simulink model "Udan_SOC"  (R2017b)
settings: Solver=FixedStepAuto  StartTime=0.0  StopTime=1000  FixedStep=0.1  RelTol=1e-3
values from neighbouring files (symbols this model uses):
  DenominatorOfIntegratorFactor = 100.0    [SOC_Stateflow.sldd]
  SOC_CalcSohLKT = 1.0    [SOC_Stateflow.sldd]
  SOC_CalcSOHTempLimit = 70.0    [SOC_Stateflow.sldd]
  SOC_CapPerCycle = 100.0    [SOC_Stateflow.sldd]
  SOC_CapTemp_HLimit = 200.0    [SOC_Stateflow.sldd]
  SOC_CapTemp_LLimit = 0.0    [SOC_Stateflow.sldd]
  Soc_ConfigInfo = 0    [SOC_Stateflow.sldd]
  SOC_DchgEndCalib = 0.0    [SOC_Stateflow.sldd]
  SOC_DiffVoltMin = 10.0    [SOC_Stateflow.sldd]
  SOC_DSOCJumpMax = 500.0    [SOC_Stateflow.sldd]
  SOC_EfficientHighLimit = 250.0    [SOC_Stateflow.sldd]
  SOC_EfficientLowLimit = 40.0    [SOC_Stateflow.sldd]
  SOC_EmptyAus = 0.0    [SOC_Stateflow.sldd]
  SOC_EnableOcv = 1.0    [SOC_Stateflow.sldd]
  SOC_END_CALIB_STATE : value not decoded    [SOC_Stateflow.sldd]
  SOC_HighRealSoc = 95.0    [SOC_Stateflow.sldd]
  SOC_LKTSohCycles = 0.0 1.0 10.0 20.0 30.0 40.0 50.0 60.0 70.0 80.0 90.0 100.0 110.0 120.0 130.0 140.0 150.0 160.0 170.0 180.0 190.0 200.0 210.0 220.0 230.0 240.0 250.0 260.0 270.0 280.0 290.0 300.0 310.0 320.0 330.0 340.0 350.0 360.0 370.0 380.0 390.0 400.0 410.0 420.0 430.0 440.0 450.0 460.0 470.0 480.0 490.0 500.0 510.0 520.0 530.0 540.0 550.0 560.0 570.0 580.0 590.0 600.0 610.0 620.0 630.0 640.0 650.0 660.0 670.0    [SOC_Stateflow.sldd]
  SOC_LKTSohTable = 1000.0 991.0 989.0 992.0 993.0 995.0 994.0 993.0 1000.0 997.0 1002.0 1000.0 992.0 1000.0 989.0 992.0 989.0 994.0 989.0 993.0 994.0 994.0 994.0 993.0 991.0 991.0 992.0 993.0 991.0 985.0 985.0 985.0 979.0 975.0 978.0 984.0 982.0 974.0 975.0 972.0 972.0 975.0 977.0 977.0 974.0 971.0 973.0 971.0 966.0 968.0 965.0 959.0 957.0 956.0 957.0 954.0 955.0 951.0 954.0 951.0 942.0 942.0 940.0 942.0 947.0 949.0    [SOC_Stateflow.sldd]
  SOC_LowRealSoc = 5.0    [SOC_Stateflow.sldd]
  SOC_NominalCap_AmS = 576000000.0    [SOC_Stateflow.sldd]
  SOC_NominalVol = 4000.0    [SOC_Stateflow.sldd]
  SOC_OCVTemp_HLimit = 106.0    [SOC_Stateflow.sldd]
  SOC_OCVTemp_LLimit = 29.0    [SOC_Stateflow.sldd]
  SOC_ShortCalibDSoc = 1.0    [SOC_Stateflow.sldd]
  SOC_SOCResolution = 10000.0    [SOC_Stateflow.sldd]
  SOC_SohCalcCapPercent = 8.0    [SOC_Stateflow.sldd]
  SOC_SohCalcHighLimit = 60.0    [SOC_Stateflow.sldd]
  SOC_SohCalcLowLimit = 10.0    [SOC_Stateflow.sldd]
  SOC_SohCalcMidLimit = 30.0    [SOC_Stateflow.sldd]
  SOC_SOHResolution = 1000.0    [SOC_Stateflow.sldd]
  SOC_State = <binary blob, 1163 chars, not shown>    [SOC_Stateflow.sldd]
  SOC_TempCap_CapBuffer : value not decoded    [SOC_Stateflow.sldd]
  SOC_TempCap_TempBuffer : value not decoded    [SOC_Stateflow.sldd]
  SocOcvCalib_ConfigInfo = 0.0    [SOC_Stateflow.sldd]
  SocOcvCalib_SocBuffer1 : value not decoded    [SOC_Stateflow.sldd]
  SocOcvCalib_TempBuffer : value not decoded    [SOC_Stateflow.sldd]
  SocOcvCalib_VoltageBuffer1 = 3300.0 3303.0 3305.0 3307.0 3310.0 3311.0 3313.0 3314.0 3316.0 3317.0 3319.0 3320.0 3322.0 3323.0 3325.0 3322.0 3323.0 3325.0 3310.0 3313.0 3315.0 3317.0 3320.0 3321.0 3323.0 3324.0 3326.0 3327.0 3329.0 3330.0 3332.0 3333.0 3335.0 3332.0 3333.0 3335.0 3320.0 3323.0 3325.0 3327.0 3330.0 3331.0 3333.0 3334.0 3336.0 3337.0 3339.0 3340.0 3342.0 3343.0 3345.0 3342.0 3343.0 3345.0 3330.0 3333.0 3335.0 3    [SOC_Stateflow.sldd]
  SOHCalibCycle = 10.0    [SOC_Stateflow.sldd]
undefined symbols (not defined in the file or in its folder): DatetimeM_GetReturnType, ParameterM_EeepParaIndexType, Soc_CumuLativeTypeType, SOC_EgthTempChgValue, Soc_EnergyBuffer, SOC_FithTempChgValue, SOC_FstSlowTempChgValue, SOC_FstTempChgValue, SOC_FthTempChgValue, SOC_MaxCap_AmS, SOC_SethTempChgValue, SOC_SixTempChgValue, SOC_SndSlowTempChgValue, SOC_SndTempChgValue, SOC_TrdSlowTempChgValue, SOC_TrdTempChgValue, SocDiagCalib_NoCalibReasonType
libraries: simulink x138, hdlsllib x24, dspindex x4
(part 7 of 10)

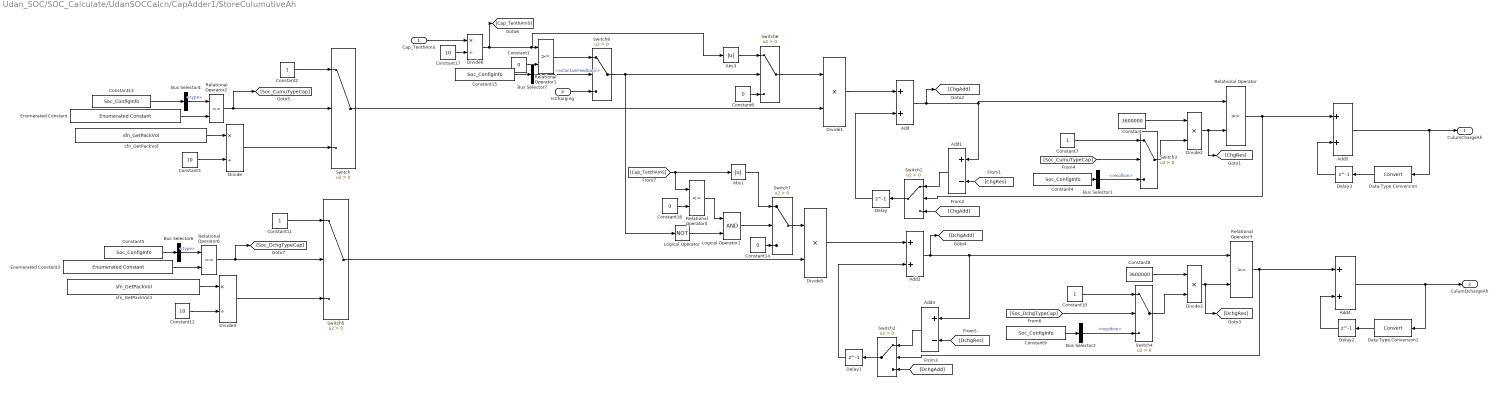
== system Udan_SOC/SOC_Calculate/UdanSOCCalcn/CapAdder1/StoreCulumutiveAh ==
  Cap_TenthAmS : Inport
  IsCharging : Inport  Port=2
  Abs1 : Abs
  Abs3 : Abs
  Add : Sum  OutDataTypeStr=uint32
  Add1 : Sum  Inputs=+-  OutDataTypeStr=int32
  Add2 : Sum  OutDataTypeStr=uint32
  Add3 : Sum  Inputs=+-  OutDataTypeStr=int32
  Add4 : Sum
  Add5 : Sum
  Bus Selector1 : BusSelector  OutputSignals=ChgCumuInfo.resoltion
  Bus Selector2 : BusSelector  OutputSignals=DchgCumuInfo.resoltion
  Bus Selector4 : BusSelector  OutputSignals=ChgCumuInfo.type
  Bus Selector6 : BusSelector  OutputSignals=DchgCumuInfo.type
  Bus Selector7 : BusSelector  OutputSignals=ChgCumuInfo.isContainFeedback
  Constant : Constant  Value=3600000  OutDataTypeStr=uint32
  Constant{1,6,14,16} (4 alike) : Constant  Value=0  OutDataTypeStr=uint8
  Constant{2,7,10..11} (4 alike) : Constant  OutDataTypeStr=uint16
  Constant12 : Constant  Value=10  OutDataTypeStr=uint8
  Constant{4..5,9,13,15} (5 alike) : Constant  Value=Soc_ConfigInfo  OutDataTypeStr=Bus: Soc_ConfigInfoType
  Constant17 : Constant  Value=10  OutDataTypeStr=uint8
  Constant3 : Constant  Value=10  OutDataTypeStr=uint8
  Constant8 : Constant  Value=3600000  OutDataTypeStr=uint32
  Data Type Conversion : DataTypeConversion
  Data Type Conversion1 : DataTypeConversion
  Delay{,1..3} (4 alike) : Delay  DelayLength=1  InitialCondition=0
  Divide : Product  Inputs=*/  OutDataTypeStr=uint16
  Divide{1..3,5} (4 alike) : Product  Inputs=**  OutDataTypeStr=uint32
  Divide4 : Product  Inputs=*/  OutDataTypeStr=uint16
  Divide6 : Product  Inputs=*/  OutDataTypeStr=int32
  Enumerated Constant : simulink/Sources/Enumerated Constant  OutDataTypeStr=Enum: Soc_CumuLativeTypeType  Value=Soc_CumuLativeTypeType.Soc_CumuTypeCap  SampleTime=inf
      settings: SourceProductName=Simulink
  Enumerated Constant3 : simulink/Sources/Enumerated Constant  OutDataTypeStr=Enum: Soc_CumuLativeTypeType  Value=Soc_CumuLativeTypeType.Soc_CumuTypeCap  SampleTime=inf
      settings: SourceProductName=Simulink
  Logical Operator : Logic  Operator=NOT  AllPortsSameDT=off  OutDataTypeStr=boolean
  Logical Operator1 : Logic  AllPortsSameDT=off  OutDataTypeStr=boolean
  Relational Operator : RelationalOperator  OutDataTypeStr=boolean  RndMeth=Simplest
  Relational Operator1 : RelationalOperator  OutDataTypeStr=boolean  RndMeth=Simplest
  Relational Operator2 : RelationalOperator  Operator===  OutDataTypeStr=boolean  RndMeth=Simplest
  Relational Operator3 : RelationalOperator  OutDataTypeStr=boolean  RndMeth=Simplest
  Relational Operator4 : RelationalOperator  Operator=<=  OutDataTypeStr=boolean  RndMeth=Simplest
  Relational Operator6 : RelationalOperator  Operator===  OutDataTypeStr=boolean  RndMeth=Simplest
  Switch{,1..2,5,8} (5 alike) : Switch  Criteria=u2 > Threshold
  Switch3 : Switch  Criteria=u2 > Threshold  OutDataTypeStr=uint16
  Switch4 : Switch  Criteria=u2 > Threshold  OutDataTypeStr=uint16
  Switch6 : Switch  Criteria=u2 > Threshold  OutDataTypeStr=uint32
  Switch7 : Switch  Criteria=u2 > Threshold  OutDataTypeStr=int32
  sfn_GetPackVol : S-Function  FunctionName=sfn_GetPackVol  SFunctionDeploymentMode=off  EnableBusSupport=off  mask(Legacy Function){SFunctionSpec=uint16 y1=Statistic_GetBcu100mvTotalVoltage(void), ShowSpec=on}
      mask prompts: ShowSpec "Display function specification"
      mask help:
      | This block allows you to call the legacy functions specified by the following Legacy Code Tool definition:
      | def.SFunctionName = 'sfn_GetPackVol';
      | def.OutputFcnSpec = 'uint16 y1=Statistic_GetBcu100mvTotalVoltage(void)';
      | def.HeaderFiles = {'Statistic.h'};
      mask Help: <p>This block was generated automatically by the Legacy Code Tool. For detailed help on this tool, call<a href="matlab:legacy_code('help')"> legacy_code('help')</a>.</p>
      mask Callback ShowSpec:
      | if strcmp(get_param(gcbh, 'ShowSpec'), 'on')
      |   set_param(gcbh, 'MaskDisplay', sprintf('fprintf(''%s'');', get_param(gcbh, 'SFunctionSpec')));
      | else
      |   set_param(gcbh, 'MaskDisplay', sprintf('fprintf(''%s'');', get_param(gcbh, 'FunctionName')));
      | end
      mask Display: fprintf('uint16 y1=Statistic_GetBcu100mvTotalVoltage(void)');
  sfn_GetPackVol1 : S-Function  FunctionName=sfn_GetPackVol  SFunctionDeploymentMode=off  EnableBusSupport=off  mask(Legacy Function){SFunctionSpec=uint16 y1=Statistic_GetBcu100mvTotalVoltage(void), ShowSpec=on}
      mask prompts: ShowSpec "Display function specification"
      mask help:
      | This block allows you to call the legacy functions specified by the following Legacy Code Tool definition:
      | def.SFunctionName = 'sfn_GetPackVol';
      | def.OutputFcnSpec = 'uint16 y1=Statistic_GetBcu100mvTotalVoltage(void)';
      | def.HeaderFiles = {'Statistic.h'};
      mask Help: <p>This block was generated automatically by the Legacy Code Tool. For detailed help on this tool, call<a href="matlab:legacy_code('help')"> legacy_code('help')</a>.</p>
      mask Callback ShowSpec:
      | if strcmp(get_param(gcbh, 'ShowSpec'), 'on')
      |   set_param(gcbh, 'MaskDisplay', sprintf('fprintf(''%s'');', get_param(gcbh, 'SFunctionSpec')));
      | else
      |   set_param(gcbh, 'MaskDisplay', sprintf('fprintf(''%s'');', get_param(gcbh, 'FunctionName')));
      | end
      mask Display: fprintf('uint16 y1=Statistic_GetBcu100mvTotalVoltage(void)');
  CulumChargeAh : Outport
  CulumDchargeAh : Outport  Port=2
  wires:
  Data Type Conversion1/1 -> Delay2/1
  Data Type Conversion/1 -> Delay3/1
  Divide1/1 -> Add/1
  Add2/1 -> [DchgAdd], Add3/1, Relational Operator3/1
  Delay1/1 -> Add2/2
  [DchgRes] -> Add3/2
  Switch2/1 -> Delay1/1
  [DchgAdd] -> Switch2/3
  Add3/1 -> Switch2/1
  Delay/1 -> Add/2
  [ChgAdd] -> Switch1/3
  Add1/1 -> Switch1/1
  [ChgRes] -> Add1/2
  Divide3/1 -> Relational Operator3/2, [DchgRes]
  Divide2/1 -> [ChgRes], Relational Operator/2
  Constant4/1 -> Bus Selector1/1
  Bus Selector1/1 -> Switch3/3  "<resoltion>"
  Switch/1 -> Divide1/2
  Divide6/1 -> Relational Operator1/1, Abs3/1, [Cap_TenthAmS]
  Divide/1 -> Switch/3
  Constant3/1 -> Divide/2
  sfn_GetPackVol/1 -> Divide/1
  Constant2/1 -> Switch/1
  Relational Operator2/1 -> Switch/2, [Soc_CumuTypeCap]
  Enumerated Constant/1 -> Relational Operator2/2
  Constant13/1 -> Bus Selector4/1
  Bus Selector4/1 -> Relational Operator2/1  "<type>"
  Constant/1 -> Divide2/1
  Add/1 -> Add1/1, Relational Operator/1, [ChgAdd]
  Switch1/1 -> Delay/1
  [Soc_CumuTypeCap] -> Switch3/2
  Constant7/1 -> Switch3/1
  Switch3/1 -> Divide2/2
  Switch4/1 -> Divide3/2
  Bus Selector2/1 -> Switch4/3  "<resoltion>"
  Constant9/1 -> Bus Selector2/1
  Constant8/1 -> Divide3/1
  [Soc_DchgTypeCap] -> Switch4/2
  Constant10/1 -> Switch4/1
  Constant11/1 -> Switch5/1
  Relational Operator6/1 -> [Soc_DchgTypeCap], Switch5/2
  Constant5/1 -> Bus Selector6/1
  Enumerated Constant3/1 -> Relational Operator6/2
  Bus Selector6/1 -> Relational Operator6/1  "<type>"
  Constant12/1 -> Divide4/2
  Divide4/1 -> Switch5/3
  sfn_GetPackVol1/1 -> Divide4/1
  [Cap_TenthAmS] -> Relational Operator4/1, Abs1/1
  Switch5/1 -> Divide5/2
  Divide5/1 -> Add2/1
  Abs1/1 -> Switch7/1
  Relational Operator3/1 -> Add4/1, Switch2/2
  IsCharging/1 -> Switch8/3
  Constant1/1 -> Relational Operator1/2
  Switch8/1 -> Switch6/2, Logical Operator/1
  Switch6/1 -> Divide1/1
  Constant6/1 -> Switch6/3
  Switch7/1 -> Divide5/1
  Logical Operator/1 -> Logical Operator1/2
  Constant14/1 -> Switch7/3
  Abs3/1 -> Switch6/1
  Add4/1 -> CulumDchargeAh/1, Data Type Conversion1/1
  Delay2/1 -> Add4/2
  Relational Operator/1 -> Add5/1, Switch1/2
  Add5/1 -> CulumChargeAh/1, Data Type Conversion/1
  Delay3/1 -> Add5/2
  Constant17/1 -> Divide6/2
  Cap_TenthAmS/1 -> Divide6/1
  Bus Selector7/1 -> Switch8/2  "<isContainFeedback>"
  Constant15/1 -> Bus Selector7/1
  Relational Operator1/1 -> Switch8/1
  Constant16/1 -> Relational Operator4/2
  Logical Operator1/1 -> Switch7/2
  Relational Operator4/1 -> Logical Operator1/1

== system Udan_SOC/SOC_Calculate/UdanSOCCalcn/CapAdder2/Function-Call Subsystem ==
  DLeftCapIn : Inport
  function : TriggerPort  VariantControl=Variant
  DLeftCapOut : Outport
  wires:
  DLeftCapIn/1 -> DLeftCapOut/1

== system Udan_SOC/SOC_Calculate/UdanSOCCalcn/ClearLeftCapWOCalib/Subsystem ==
  data : Inport
  HighIndex : Inport  Port=2
  LowIndex : Inport  Port=3
  Bit Rotate : hdlsllib/Logic and Bit Operations/Bit Rotate  mode=Rotate Right  N=16
      settings: SourceProductName=HDL Coder  SourceProductBaseCode=HD
  Data Type Conversion : DataTypeConversion  OutDataTypeStr=uint16
  Data Type Conversion1 : DataTypeConversion  OutDataTypeStr=uint16
  S-Function : S-Function  FunctionName=sfn_NVMWrite  SFunctionDeploymentMode=off  EnableBusSupport=off
  S-Function1 : S-Function  FunctionName=sfn_NVMWrite  SFunctionDeploymentMode=off  EnableBusSupport=off
  Terminator : Terminator
  Terminator1 : Terminator
  wires:
  data/1 -> Data Type Conversion1/1, Bit Rotate/1
  Data Type Conversion/1 -> S-Function/2
  S-Function1/1 -> Terminator1/1
  Bit Rotate/1 -> Data Type Conversion/1
  Data Type Conversion1/1 -> S-Function1/2
  S-Function/1 -> Terminator/1
  HighIndex/1 -> S-Function/1
  LowIndex/1 -> S-Function1/1

== system Udan_SOC/SOC_Calculate/UdanSOCCalcn/ClearLeftCapWOCalib2/Subsystem ==
  data : Inport
  HighIndex : Inport  Port=2
  LowIndex : Inport  Port=3
  Bit Rotate : hdlsllib/Logic and Bit Operations/Bit Rotate  mode=Rotate Right  N=16
      settings: SourceProductName=HDL Coder  SourceProductBaseCode=HD
  Data Type Conversion : DataTypeConversion  OutDataTypeStr=uint16
  Data Type Conversion1 : DataTypeConversion  OutDataTypeStr=uint16
  S-Function : S-Function  FunctionName=sfn_NVMWrite  SFunctionDeploymentMode=off  EnableBusSupport=off
  S-Function1 : S-Function  FunctionName=sfn_NVMWrite  SFunctionDeploymentMode=off  EnableBusSupport=off
  Terminator : Terminator
  Terminator1 : Terminator
  wires:
  data/1 -> Data Type Conversion1/1, Bit Rotate/1
  Data Type Conversion/1 -> S-Function/2
  S-Function1/1 -> Terminator1/1
  Bit Rotate/1 -> Data Type Conversion/1
  Data Type Conversion1/1 -> S-Function1/2
  S-Function/1 -> Terminator/1
  HighIndex/1 -> S-Function/1
  LowIndex/1 -> S-Function1/1

== system Udan_SOC/SOC_Calculate/UdanSOCCalcn/Function-Call Subsystem/Subsystem ==
  data : Inport
  HighIndex : Inport  Port=2
  LowIndex : Inport  Port=3
  Bit Rotate : hdlsllib/Logic and Bit Operations/Bit Rotate  mode=Rotate Right  N=16
      settings: SourceProductName=HDL Coder  SourceProductBaseCode=HD
  Data Type Conversion : DataTypeConversion  OutDataTypeStr=uint16
  Data Type Conversion1 : DataTypeConversion  OutDataTypeStr=uint16
  S-Function : S-Function  FunctionName=sfn_NVMWrite  SFunctionDeploymentMode=off  EnableBusSupport=off
  S-Function1 : S-Function  FunctionName=sfn_NVMWrite  SFunctionDeploymentMode=off  EnableBusSupport=off
  Terminator : Terminator
  Terminator1 : Terminator
  wires:
  data/1 -> Data Type Conversion1/1, Bit Rotate/1
  Data Type Conversion/1 -> S-Function/2
  S-Function1/1 -> Terminator1/1
  Bit Rotate/1 -> Data Type Conversion/1
  Data Type Conversion1/1 -> S-Function1/2
  S-Function/1 -> Terminator/1
  HighIndex/1 -> S-Function/1
  LowIndex/1 -> S-Function1/1

== system Udan_SOC/SOC_Calculate/UdanSOCCalcn/Function-Call Subsystem4/Enabled Subsystem ==
  Index : Inport
  RealSoc : Inport  Port=2
  Enable : EnablePort
  S-Function1 : S-Function  FunctionName=sfn_NVMRead  SFunctionDeploymentMode=off  EnableBusSupport=off
  Switch : Switch  Criteria=u2 > Threshold
  ReadDsocAgain : Outport
  wires:
  Index/1 -> S-Function1/1
  S-Function1/1 -> Switch/2
  RealSoc/1 -> Switch/1
  S-Function1/2 -> Switch/3
  Switch/1 -> ReadDsocAgain/1

== system Udan_SOC/SOC_Calculate/UdanSOCCalcn/Function-Call Subsystem4/Enabled Subsystem1 ==
  Enable : EnablePort
  Constant2 : Constant  Value=0  OutDataTypeStr=uint8
  Constant4 : Constant  Value=SOC_SOHResolution  OutDataTypeStr=uint16
  Enumerated Constant2 : simulink/Sources/Enumerated Constant  OutDataTypeStr=Enum: ParameterM_EeepParaIndexType  Value=ParameterM_EeepParaIndexType.PARAMETERM_EEEP_SOH_INDEX  SampleTime=inf
      settings: SourceProductName=Simulink
  Relational Operator1 : RelationalOperator  Operator=~=  OutDataTypeStr=boolean  RndMeth=Simplest
  S-Function : S-Function  FunctionName=sfn_NVMRead  SFunctionDeploymentMode=off  EnableBusSupport=off
  Switch : Switch  Criteria=u2 > Threshold
  ReadAgain : Outport
  wires:
  Enumerated Constant2/1 -> S-Function/1
  Constant2/1 -> Relational Operator1/2
  S-Function/1 -> Relational Operator1/1
  Relational Operator1/1 -> Switch/2
  S-Function/2 -> Switch/3
  Switch/1 -> ReadAgain/1
  Constant4/1 -> Switch/1

== system Udan_SOC/SOC_Calculate/UdanSOCCalcn/Function-Call Subsystem4/Subsystem1 ==
  HighIndex : Inport
  LowIndex : Inport  Port=2
  DefaultValue : Inport  Port=3
  Constant1 : Constant  Value=0  OutDataTypeStr=uint8
  Constant2 : Constant  Value=0  OutDataTypeStr=uint8
  Logical Operator : Logic  AllPortsSameDT=off  OutDataTypeStr=boolean
  Logical Operator1 : Logic  Operator=NOT  AllPortsSameDT=off  OutDataTypeStr=boolean
  Relational Operator : RelationalOperator  Operator===  OutDataTypeStr=boolean  RndMeth=Simplest
  Relational Operator1 : RelationalOperator  Operator===  OutDataTypeStr=boolean  RndMeth=Simplest
  S-Function : S-Function  FunctionName=sfn_NVMRead  SFunctionDeploymentMode=off  EnableBusSupport=off
  S-Function1 : S-Function  FunctionName=sfn_NVMRead  SFunctionDeploymentMode=off  EnableBusSupport=off
  Subsystem : Subsystem
  Subsystem1 : Subsystem  mask(ReadEeep_uint32){}
  Switch : Switch  Criteria=u2 > Threshold
  EeepRead32 : Outport
  wires:
  DefaultValue/1 -> Subsystem1/3(DefaultValue)
  [ReadLowOk] -> Logical Operator/1
  S-Function/2 -> Subsystem/1(HighIndex)
  S-Function/1 -> Relational Operator/1
  S-Function1/2 -> Subsystem/2(LowIndex)
  HighIndex/1 -> [HighIndex], S-Function/1
  Constant1/1 -> Relational Operator/2
  Constant2/1 -> Relational Operator1/2
  LowIndex/1 -> [LowIndex], S-Function1/1
  Relational Operator/1 -> Logical Operator/2
  Logical Operator/1 -> Subsystem/Enable, Logical Operator1/1
  Relational Operator1/1 -> [ReadLowOk]
  S-Function1/1 -> Relational Operator1/1
  Subsystem/1(soc) -> Switch/3
  Switch/1 -> EeepRead32/1
  [HighIndex] -> Subsystem1/1(HighIndex)
  [LowIndex] -> Subsystem1/2(LowIndex)
  Logical Operator1/1 -> [Enable], Subsystem1/Enable
  Subsystem1/1(EeepRead32) -> Switch/1
  [Enable] -> Switch/2

== system Udan_SOC/SOC_Calculate/UdanSOCCalcn/Function-Call Subsystem4/Subsystem2 ==
  SOH : Inport
  Enable : EnablePort
  Bus Selector2 : BusSelector  OutputSignals=DchgCumuInfo.resoltion
  Bus Selector4 : BusSelector  OutputSignals=DchgCumuInfo.type
  Constant : Constant  Value=SOC_LKTSohTable  VectorParams1D=off
  Constant1 : Constant  Value=SOC_LKTSohCycles  VectorParams1D=off
  Constant16 : Constant  Value=SOC_NominalCap_AmS
  Constant17 : Constant  Value=3600000  OutDataTypeStr=uint32
  Constant25 : Constant  Value=Soc_ConfigInfo  OutDataTypeStr=Bus: Soc_ConfigInfoType
  Constant26 : Constant  Value=10  OutDataTypeStr=uint8
  Constant27 : Constant  Value=Soc_ConfigInfo  OutDataTypeStr=Bus: Soc_ConfigInfoType
  Constant28 : Constant  Value=SOC_NominalVol
  Constant29 : Constant  Value=SOC_NominalCap_AmS
  Constant30 : Constant  Value=3600000  OutDataTypeStr=uint32
  Constant31 : Constant  Value=SOC_CapPerCycle  OutDataTypeStr=uint8
  Constant32 : Constant  Value=100  OutDataTypeStr=uint8
  Constant4 : Constant  Value=SOC_CapPerCycle  OutDataTypeStr=uint8
  Constant5 : Constant  Value=100  OutDataTypeStr=uint8
  DchgPower1 : simulink/Sources/Enumerated Constant  OutDataTypeStr=Enum: ParameterM_EeepParaIndexType  Value=ParameterM_EeepParaIndexType.PARAMETERM_EEEP_CUMULATIVE_DCHG_CAP_L_INDEX  SampleTime=inf
      settings: SourceProductName=Simulink
  DchgPower2 : simulink/Sources/Enumerated Constant  OutDataTypeStr=Enum: ParameterM_EeepParaIndexType  Value=ParameterM_EeepParaIndexType.PARAMETERM_EEEP_CUMULATIVE_DCHG_CAP_H_INDEX  SampleTime=inf
      settings: SourceProductName=Simulink
  Divide1 : Product  Inputs=*/*/  OutDataTypeStr=uint32
  Divide11 : Product  Inputs=**  OutDataTypeStr=uint32
  Divide6 : Product  Inputs=*/*/  OutDataTypeStr=uint32
  Divide7 : Product  Inputs=**//  OutDataTypeStr=uint32  RndMeth=Round
  Enumerated Constant8 : simulink/Sources/Enumerated Constant  OutDataTypeStr=Enum: Soc_CumuLativeTypeType  Value=Soc_CumuLativeTypeType.Soc_CumuTypeCap  SampleTime=inf
      settings: SourceProductName=Simulink
  MATLAB Function2 : MATLAB Function  TreatAsAtomicUnit=on
  MATLAB Function3 : MATLAB Function  TreatAsAtomicUnit=on
  Relational Operator12 : RelationalOperator  Operator===  OutDataTypeStr=boolean  RndMeth=Simplest
  Subsystem : Subsystem  mask(EeepWrite_uint32){}
      mask help: EeepWrite_uint32
  Switch7 : Switch  Criteria=u2 > Threshold
  wires:
  MATLAB Function2/1(y) -> Divide11/1
  Divide11/1 -> Subsystem/1(data)
  DchgPower2/1 -> Subsystem/2(HighIndex)
  DchgPower1/1 -> Subsystem/3(LowIndex)
  SOH/1 -> MATLAB Function3/1(soh), MATLAB Function2/1(input)
  Constant/1 -> MATLAB Function3/3(Table)
  MATLAB Function3/1(bp) -> MATLAB Function2/2(bp)
  MATLAB Function3/2(table) -> MATLAB Function2/3(table)
  Constant1/1 -> MATLAB Function3/2(Cycles)
  Divide7/1 -> Switch7/3
  Switch7/1 -> Divide11/2
  Relational Operator12/1 -> Switch7/2
  Constant30/1 -> Divide6/2
  Divide1/1 -> Switch7/1
  Constant29/1 -> Divide6/1
  Constant17/1 -> Divide1/2
  Divide6/1 -> Divide7/1
  Constant26/1 -> Divide7/3
  Constant32/1 -> Divide6/4
  Constant27/1 -> Bus Selector2/1
  Constant28/1 -> Divide7/2
  Bus Selector2/1 -> Divide7/4  "<resoltion>"
  Enumerated Constant8/1 -> Relational Operator12/2
  Constant31/1 -> Divide6/3
  Constant4/1 -> Divide1/3
  Constant25/1 -> Bus Selector4/1
  Constant5/1 -> Divide1/4
  Constant16/1 -> Divide1/1
  Bus Selector4/1 -> Relational Operator12/1  "<type>"

== system Udan_SOC/SOC_Calculate/UdanSOCCalcn/LKTSOC/CalcLeftCap ==
  soc : Inport
  LookUpTempCap : Inport  Port=2
  SOH : Inport  Port=3
  Enable : EnablePort
  Abs : Abs
  Add : Sum  OutDataTypeStr=uint32
  Add1 : Sum  Inputs=+-  OutDataTypeStr=int32
  Bus Creator1 : BusCreator  Inputs=2  OutDataTypeStr=Bus: Capacity
      settings: InheritFromInputs=off
  Constant1 : Constant  Value=0  OutDataTypeStr=int32
  Constant10 : Constant  Value=SOC_SOCResolution  OutDataTypeStr=uint16
  Constant2 : Constant  Value=0  OutDataTypeStr=uint16
  Constant3 : Constant  Value=0  OutDataTypeStr=uint32
  Constant5 : Constant  Value=SOC_NominalCap_AmS
  Constant6 : Constant  Value=SOC_NominalCap_AmS
  Constant8 : Constant  Value=SOC_SOHResolution  OutDataTypeStr=uint16
  Constant9 : Constant  Value=2  OutDataTypeStr=uint8
  Divide : Product  Inputs=*/*  OutDataTypeStr=uint32
  Divide1 : Product  Inputs=*/*  OutDataTypeStr=uint32
  Divide4 : Product  Inputs=**  OutDataTypeStr=uint32
  Saturation Dynamic : simulink/Discontinuities/Saturation Dynamic  OutMin=[]  OutMax=[]  OutDataTypeStr=Inherit: Same as second input  OutDataType=fixdt(1, 16)  OutScaling=2^-10  DoSatur=off
  Switch : Switch  Criteria=u2 > Threshold  OutDataTypeStr=int32
  LeftCap : Outport
  wires:
  Divide1/1 -> Saturation Dynamic/2
  soc/1 -> Divide/3
  Constant10/1 -> Divide/2
  Add/1 -> Divide1/1
  Saturation Dynamic/1 -> Bus Creator1/1  "AmS"
  Constant2/1 -> Saturation Dynamic/3
  Divide/1 -> Add/1
  Constant5/1 -> Add1/2
  Divide4/1 -> Saturation Dynamic/1
  LookUpTempCap/1 -> Add1/1, Divide/1
  Constant8/1 -> Divide1/2
  Bus Creator1/1 -> LeftCap/1
  Switch/1 -> Abs/1
  Abs/1 -> Add/2
  Add1/1 -> Switch/3, Switch/2
  Constant3/1 -> Switch/1
  Constant1/1 -> Bus Creator1/2  "AuS"
  Constant6/1 -> Divide4/1
  Constant9/1 -> Divide4/2
  SOH/1 -> Divide1/3

== system Udan_SOC/SOC_Calculate/UdanSOCCalcn/LKTSOC/Subsystem ==
  SOC_LeftCap0 : Inport
  SOC_LeftCap2 : Inport  Port=2
  SOHIn : Inport  Port=3
  WOCalibAh : Inport  Port=4
  Enable : EnablePort
  Chart1 : Stateflow chart  TreatAsAtomicUnit=on
  Constant1 : Constant  Value=1200  OutDataTypeStr=uint16
  Constant10 : Constant  Value=65535  OutDataTypeStr=uint16
  Constant2 : Constant  Value=800  OutDataTypeStr=uint16
  Constant3 : Constant  Value=SOC_SohCalcHighLimit
  Constant31 : Constant  Value=SOC_NominalCap_AmS
  Constant4 : Constant  Value=1000  OutDataTypeStr=uint16
  Constant5 : Constant  Value=SOC_SohCalcLowLimit
  Constant6 : Constant  Value=SOC_SohCalcMidLimit
  Constant7 : Constant  Value=SOC_SOCResolution  OutDataTypeStr=uint16
  Constant8 : Constant  Value=1000  OutDataTypeStr=uint16
  Constant9 : Constant  Value=1000  OutDataTypeStr=uint16
  DchgPower1 : simulink/Sources/Enumerated Constant  OutDataTypeStr=Enum: ParameterM_EeepParaIndexType  Value=ParameterM_EeepParaIndexType.PARAMETERM_EEEP_SOH_Full_INDEX  SampleTime=inf
      settings: SourceProductName=Simulink
  Divide : Product  Inputs=**  OutDataTypeStr=uint32
  Divide1 : Product  Inputs=*/  OutDataTypeStr=uint32
  Divide2 : Product  Inputs=*/  OutDataTypeStr=uint32
  Divide3 : Product  Inputs=*/  OutDataTypeStr=uint32
  Divide4 : Product  Inputs=*/*  OutDataTypeStr=uint32
  Relational Operator : RelationalOperator  Operator=~=  OutDataTypeStr=boolean  RndMeth=Simplest
  S-Function1 : S-Function  FunctionName=sfn_NVMWrite  SFunctionDeploymentMode=off  EnableBusSupport=off
  Saturation Dynamic : simulink/Discontinuities/Saturation Dynamic  OutMin=[]  OutMax=[]  OutDataTypeStr=Inherit: Same as second input  OutDataType=fixdt(1, 16)  OutScaling=2^-10  DoSatur=off
  Subtract2 : Sum  Inputs=+-
  Switch : Switch  Criteria=u2 > Threshold
  Terminator : Terminator
  Terminator1 : Terminator
  SohOut : Outport
  wires:
  Divide2/1 -> Saturation Dynamic/2
  Chart1/1(SOHWriteResult) -> Terminator/1
  Constant2/1 -> Saturation Dynamic/3
  Constant4/1 -> Divide3/2
  SOC_LeftCap2/1 -> Switch/1, Relational Operator/1
  Divide3/1 -> Divide2/2
  Saturation Dynamic/1 -> Chart1/1(CalcSOH)
  Chart1/2(SohOut) -> SohOut/1
  SOHIn/1 -> [SOHIn], Divide4/3
  Subtract2/1 -> Divide3/1
  Constant1/1 -> Saturation Dynamic/1
  SOC_LeftCap0/1 -> Divide/1
  WOCalibAh/1 -> Divide4/1
  Constant7/1 -> Divide1/2
  Divide1/1 -> Divide/2
  Constant31/1 -> Divide1/1
  Divide/1 -> Relational Operator/2, Subtract2/1
  Relational Operator/1 -> Switch/2
  Constant8/1 -> Switch/3
  Switch/1 -> Subtract2/2
  Constant9/1 -> Divide4/2
  Divide4/1 -> Divide2/1
  [SOHIn] -> Chart1/5(EEEPSOH)
  S-Function1/1 -> Terminator1/1
  Constant10/1 -> S-Function1/2
  DchgPower1/1 -> S-Function1/1
  Constant3/1 -> Chart1/2(MaxDiff)
  Constant6/1 -> Chart1/3(MaxCal)
  Constant5/1 -> Chart1/4(MaxCal1)

== system Udan_SOC/SOC_Calculate/UdanSOCCalcn/LKTSOC/Subsystem1 ==
  HighIndex : Inport
  LowIndex : Inport  Port=2
  DefaultValue : Inport  Port=3
  Constant1 : Constant  Value=0  OutDataTypeStr=uint8
  Constant2 : Constant  Value=0  OutDataTypeStr=uint8
  Logical Operator : Logic  AllPortsSameDT=off  OutDataTypeStr=boolean
  Logical Operator1 : Logic  Operator=NOT  AllPortsSameDT=off  OutDataTypeStr=boolean
  Relational Operator : RelationalOperator  Operator===  OutDataTypeStr=boolean  RndMeth=Simplest
  Relational Operator1 : RelationalOperator  Operator===  OutDataTypeStr=boolean  RndMeth=Simplest
  S-Function : S-Function  FunctionName=sfn_NVMRead  SFunctionDeploymentMode=off  EnableBusSupport=off
  S-Function1 : S-Function  FunctionName=sfn_NVMRead  SFunctionDeploymentMode=off  EnableBusSupport=off
  Subsystem : Subsystem
  Switch : Switch  Criteria=u2 > Threshold
  EeepRead32 : Outport
  wires:
  DefaultValue/1 -> Switch/1
  [ReadLowOk] -> Logical Operator/1
  S-Function/2 -> Subsystem/1(HighIndex)
  S-Function/1 -> Relational Operator/1
  S-Function1/2 -> Subsystem/2(LowIndex)
  HighIndex/1 -> S-Function/1
  Constant1/1 -> Relational Operator/2
  Constant2/1 -> Relational Operator1/2
  LowIndex/1 -> S-Function1/1
  Relational Operator/1 -> Logical Operator/2
  Logical Operator/1 -> Logical Operator1/1, Subsystem/Enable
  Relational Operator1/1 -> [ReadLowOk]
  S-Function1/1 -> Relational Operator1/1
  Subsystem/1(soc) -> Switch/3
  Logical Operator1/1 -> Switch/2
  Switch/1 -> EeepRead32/1

== system Udan_SOC/SOC_Calculate/UdanSOCCalcn/SetSOHCalcFlag/Subsystem ==
  data : Inport
  HighIndex : Inport  Port=2
  LowIndex : Inport  Port=3
  Bit Rotate : hdlsllib/Logic and Bit Operations/Bit Rotate  mode=Rotate Right  N=16
      settings: SourceProductName=HDL Coder  SourceProductBaseCode=HD
  Data Type Conversion : DataTypeConversion  OutDataTypeStr=uint16
  Data Type Conversion1 : DataTypeConversion  OutDataTypeStr=uint16
  S-Function : S-Function  FunctionName=sfn_NVMWrite  SFunctionDeploymentMode=off  EnableBusSupport=off
  S-Function1 : S-Function  FunctionName=sfn_NVMWrite  SFunctionDeploymentMode=off  EnableBusSupport=off
  Terminator : Terminator
  Terminator1 : Terminator
  wires:
  data/1 -> Data Type Conversion1/1, Bit Rotate/1
  Data Type Conversion/1 -> S-Function/2
  S-Function1/1 -> Terminator1/1
  Bit Rotate/1 -> Data Type Conversion/1
  Data Type Conversion1/1 -> S-Function1/2
  S-Function/1 -> Terminator/1
  HighIndex/1 -> S-Function/1
  LowIndex/1 -> S-Function1/1

== system Udan_SOC/SOC_Calculate/UdanSOCCalcn/SetSOHCalcFlagFullChg/Subsystem ==
  data : Inport
  HighIndex : Inport  Port=2
  LowIndex : Inport  Port=3
  Bit Rotate : hdlsllib/Logic and Bit Operations/Bit Rotate  mode=Rotate Right  N=16
      settings: SourceProductName=HDL Coder  SourceProductBaseCode=HD
  Data Type Conversion : DataTypeConversion  OutDataTypeStr=uint16
  Data Type Conversion1 : DataTypeConversion  OutDataTypeStr=uint16
  S-Function : S-Function  FunctionName=sfn_NVMWrite  SFunctionDeploymentMode=off  EnableBusSupport=off
  S-Function1 : S-Function  FunctionName=sfn_NVMWrite  SFunctionDeploymentMode=off  EnableBusSupport=off
  Terminator : Terminator
  Terminator1 : Terminator
  wires:
  data/1 -> Data Type Conversion1/1, Bit Rotate/1
  Data Type Conversion/1 -> S-Function/2
  S-Function1/1 -> Terminator1/1
  Bit Rotate/1 -> Data Type Conversion/1
  Data Type Conversion1/1 -> S-Function1/2
  S-Function/1 -> Terminator/1
  HighIndex/1 -> S-Function/1
  LowIndex/1 -> S-Function1/1

== system Udan_SOC/SOC_Calculate/UdanSOCCalcn/StoreCulumutiveAh/StoreChgAh ==
  Enable : EnablePort
  Add : Sum  OutDataTypeStr=uint32
  Bus Selector4 : BusSelector  OutputSignals=ChgCumuInfo.type
  Constant1 : Constant  Value=0  OutDataTypeStr=uint32
  Constant13 : Constant  Value=Soc_ConfigInfo  OutDataTypeStr=Bus: Soc_ConfigInfoType
  Constant2 : Constant  OutDataTypeStr=uint16
  Constant7 : Constant  OutDataTypeStr=uint16
  DchgPower1 : simulink/Sources/Enumerated Constant  OutDataTypeStr=Enum: ParameterM_EeepParaIndexType  Value=ParameterM_EeepParaIndexType.PARAMETERM_EEEP_CUMULATIVE_CHG_CAP_L_INDEX  SampleTime=inf
      settings: SourceProductName=Simulink
  DchgPower2 : simulink/Sources/Enumerated Constant  OutDataTypeStr=Enum: ParameterM_EeepParaIndexType  Value=ParameterM_EeepParaIndexType.PARAMETERM_EEEP_CUMULATIVE_CHG_CAP_H_INDEX  SampleTime=inf
      settings: SourceProductName=Simulink
  DchgPower3 : simulink/Sources/Enumerated Constant  OutDataTypeStr=Enum: ParameterM_EeepParaIndexType  Value=ParameterM_EeepParaIndexType.PARAMETERM_EEEP_CUMULATIVE_CHG_CAP_H_INDEX  SampleTime=inf
      settings: SourceProductName=Simulink
  DchgPower4 : simulink/Sources/Enumerated Constant  OutDataTypeStr=Enum: ParameterM_EeepParaIndexType  Value=ParameterM_EeepParaIndexType.PARAMETERM_EEEP_CUMULATIVE_CHG_CAP_L_INDEX  SampleTime=inf
      settings: SourceProductName=Simulink
  Enumerated Constant : simulink/Sources/Enumerated Constant  OutDataTypeStr=Enum: Soc_CumuLativeTypeType  Value=Soc_CumuLativeTypeType.Soc_CumuTypeCap  SampleTime=inf
      settings: SourceProductName=Simulink
  Relational Operator2 : RelationalOperator  Operator===  OutDataTypeStr=boolean  RndMeth=Simplest
  Subsystem : Subsystem  mask(EeepWrite_uint32){}
      mask help: EeepWrite_uint32
  Subsystem1 : Subsystem  mask(ReadEeep_uint32){}
  Switch3 : Switch  Criteria=u2 > Threshold  OutDataTypeStr=uint16
  wires:
  DchgPower4/1 -> Subsystem/3(LowIndex)
  DchgPower3/1 -> Subsystem/2(HighIndex)
  Add/1 -> Subsystem/1(data)
  DchgPower2/1 -> Subsystem1/1(HighIndex)
  DchgPower1/1 -> Subsystem1/2(LowIndex)
  Subsystem1/1(EeepRead32) -> Add/1
  Constant1/1 -> Subsystem1/3(DefaultValue)
  Switch3/1 -> Add/2
  Constant2/1 -> Switch3/3
  Constant7/1 -> Switch3/1
  Relational Operator2/1 -> Switch3/2
  Enumerated Constant/1 -> Relational Operator2/2
  Bus Selector4/1 -> Relational Operator2/1  "<type>"
  Constant13/1 -> Bus Selector4/1

== system Udan_SOC/SOC_Calculate/UdanSOCCalcn/StoreCulumutiveAh/StoreDchgAh1 ==
  Enable : EnablePort
  Add : Sum  OutDataTypeStr=uint32
  Bus Selector3 : BusSelector  OutputSignals=DchgCumuInfo.type
  Constant1 : Constant  Value=0  OutDataTypeStr=uint32
  Constant10 : Constant  OutDataTypeStr=uint16
  Constant2 : Constant  Value=Soc_ConfigInfo  OutDataTypeStr=Bus: Soc_ConfigInfoType
  Constant3 : Constant  OutDataTypeStr=uint16
  DchgPower1 : simulink/Sources/Enumerated Constant  OutDataTypeStr=Enum: ParameterM_EeepParaIndexType  Value=ParameterM_EeepParaIndexType.PARAMETERM_EEEP_CUMULATIVE_DCHG_CAP_L_INDEX  SampleTime=inf
      settings: SourceProductName=Simulink
  DchgPower2 : simulink/Sources/Enumerated Constant  OutDataTypeStr=Enum: ParameterM_EeepParaIndexType  Value=ParameterM_EeepParaIndexType.PARAMETERM_EEEP_CUMULATIVE_DCHG_CAP_H_INDEX  SampleTime=inf
      settings: SourceProductName=Simulink
  DchgPower3 : simulink/Sources/Enumerated Constant  OutDataTypeStr=Enum: ParameterM_EeepParaIndexType  Value=ParameterM_EeepParaIndexType.PARAMETERM_EEEP_CUMULATIVE_DCHG_CAP_H_INDEX  SampleTime=inf
      settings: SourceProductName=Simulink
  DchgPower4 : simulink/Sources/Enumerated Constant  OutDataTypeStr=Enum: ParameterM_EeepParaIndexType  Value=ParameterM_EeepParaIndexType.PARAMETERM_EEEP_CUMULATIVE_DCHG_CAP_L_INDEX  SampleTime=inf
      settings: SourceProductName=Simulink
  Enumerated Constant2 : simulink/Sources/Enumerated Constant  OutDataTypeStr=Enum: Soc_CumuLativeTypeType  Value=Soc_CumuLativeTypeType.Soc_CumuTypeCap  SampleTime=inf
      settings: SourceProductName=Simulink
  Relational Operator4 : RelationalOperator  Operator===  OutDataTypeStr=boolean  RndMeth=Simplest
  Subsystem : Subsystem  mask(EeepWrite_uint32){}
      mask help: EeepWrite_uint32
  Subsystem1 : Subsystem  mask(ReadEeep_uint32){}
  Switch4 : Switch  Criteria=u2 > Threshold  OutDataTypeStr=uint16
  wires:
  DchgPower4/1 -> Subsystem/3(LowIndex)
  DchgPower3/1 -> Subsystem/2(HighIndex)
  Add/1 -> Subsystem/1(data)
  DchgPower2/1 -> Subsystem1/1(HighIndex)
  DchgPower1/1 -> Subsystem1/2(LowIndex)
  Subsystem1/1(EeepRead32) -> Add/1
  Constant1/1 -> Subsystem1/3(DefaultValue)
  Enumerated Constant2/1 -> Relational Operator4/2
  Constant10/1 -> Switch4/1
  Bus Selector3/1 -> Relational Operator4/1  "<type>"
  Constant2/1 -> Bus Selector3/1
  Relational Operator4/1 -> Switch4/2
  Switch4/1 -> Add/2
  Constant3/1 -> Switch4/3

== system Udan_SOC/SOC_Calculate/UdanSOCCalcn/StoreDSOC/WriteLeftCap ==
  DSOC : Inport
  Enable : EnablePort
  Data Type Conversion : DataTypeConversion  OutDataTypeStr=uint16
  Enumerated Constant : simulink/Sources/Enumerated Constant  OutDataTypeStr=Enum: ParameterM_EeepParaIndexType  Value=ParameterM_EeepParaIndexType.PARAMETERM_EEEP_MODEL_DSOC_INDEX  SampleTime=inf
      settings: SourceProductName=Simulink
  S-Function : S-Function  FunctionName=sfn_NVMWrite  SFunctionDeploymentMode=off  EnableBusSupport=off
  Terminator : Terminator
  wires:
  Enumerated Constant/1 -> S-Function/1
  DSOC/1 -> Data Type Conversion/1
  Data Type Conversion/1 -> S-Function/2
  S-Function/1 -> Terminator/1

== system Udan_SOC/SOC_Calculate/UdanSOCCalcn/StoreLeftCap/WriteLeftCap ==
  cap : Inport
  Enable : EnablePort
  Enumerated Constant : simulink/Sources/Enumerated Constant  OutDataTypeStr=Enum: ParameterM_EeepParaIndexType  Value=ParameterM_EeepParaIndexType.PARAMETERM_EEEP_LEFTCAP_H_INDEX  SampleTime=inf
      settings: SourceProductName=Simulink
  Enumerated Constant1 : simulink/Sources/Enumerated Constant  OutDataTypeStr=Enum: ParameterM_EeepParaIndexType  Value=ParameterM_EeepParaIndexType.PARAMETERM_EEEP_LEFTCAP_L_INDEX  SampleTime=inf
      settings: SourceProductName=Simulink
  Subsystem : Subsystem  mask(EeepWrite_uint32){}
      mask help: EeepWrite_uint32
  wires:
  Enumerated Constant1/1 -> Subsystem/3(LowIndex)
  Enumerated Constant/1 -> Subsystem/2(HighIndex)
  cap/1 -> Subsystem/1(data)

== system Udan_SOC/SOC_Calculate/UdanSOCCalcn/StoreSOC/Subsystem ==
  CurrentAmS : Inport
  Enable : EnablePort
  Abs : Abs
  Add1 : Sum  OutDataTypeStr=uint32
  Add2 : Sum  Inputs=+-  OutDataTypeStr=int32
  Constant16 : Constant  Value=SOC_NominalCap_AmS
  Constant5 : Constant  Value=35  OutDataTypeStr=uint8
  Delay1 : Delay  DelayLength=1  InitialCondition=0
  Divide8 : Product  Inputs=*/  OutDataTypeStr=uint32
  Enabled Subsystem1 : Subsystem  TreatAsAtomicUnit=on
  Logical Operator : Logic  Operator=NOT  AllPortsSameDT=off  OutDataTypeStr=boolean
  Logical Operator1 : Logic  Operator=OR  Inputs=1  AllPortsSameDT=off  OutDataTypeStr=boolean
  Relational Operator : RelationalOperator  Operator=<=  OutDataTypeStr=boolean  RndMeth=Nearest
  Switch : Switch  Criteria=u2 > Threshold
  wires:
  CurrentAmS/1 -> Abs/1
  Abs/1 -> Add1/2
  Add1/1 -> Add2/1, Switch/1, Relational Operator/1
  Add2/1 -> Switch/3
  Relational Operator/1 -> Switch/2, Logical Operator/1
  Switch/1 -> Delay1/1
  Delay1/1 -> Add1/1
  Logical Operator/1 -> Logical Operator1/1
  Logical Operator1/1 -> Enabled Subsystem1/Enable
  Divide8/1 -> Relational Operator/2, Add2/2
  Constant16/1 -> Divide8/1
  Constant5/1 -> Divide8/2

== system Udan_SOC/SOC_Calculate/UdanSOCCalcn/StoreSOC/Subsystem1 ==
  CurrentAmS : Inport
  Enable : EnablePort
  Abs : Abs
  Add1 : Sum  OutDataTypeStr=uint32
  Add2 : Sum  Inputs=+-  OutDataTypeStr=int32
  Constant16 : Constant  Value=SOC_NominalCap_AmS
  Constant5 : Constant  Value=35  OutDataTypeStr=uint8
  Delay1 : Delay  DelayLength=1  InitialCondition=0
  Divide8 : Product  Inputs=*/  OutDataTypeStr=uint32
  Enabled Subsystem1 : Subsystem  TreatAsAtomicUnit=on
  Logical Operator : Logic  Operator=NOT  AllPortsSameDT=off  OutDataTypeStr=boolean
  Logical Operator1 : Logic  Operator=OR  Inputs=1  AllPortsSameDT=off  OutDataTypeStr=boolean
  Relational Operator : RelationalOperator  Operator=<=  OutDataTypeStr=boolean  RndMeth=Nearest
  Switch : Switch  Criteria=u2 > Threshold
  wires:
  CurrentAmS/1 -> Abs/1
  Abs/1 -> Add1/2
  Add1/1 -> Add2/1, Switch/1, Relational Operator/1
  Add2/1 -> Switch/3
  Relational Operator/1 -> Switch/2, Logical Operator/1
  Switch/1 -> Delay1/1
  Delay1/1 -> Add1/1
  Logical Operator/1 -> Logical Operator1/1
  Logical Operator1/1 -> Enabled Subsystem1/Enable
  Divide8/1 -> Relational Operator/2, Add2/2
  Constant5/1 -> Divide8/2
  Constant16/1 -> Divide8/1

== system Udan_SOC/SOC_Calculate/UdanSOCCalcn/StoreTSOC/WriteLeftCap ==
  DSOC : Inport
  Enable : EnablePort
  Data Type Conversion : DataTypeConversion  OutDataTypeStr=uint16
  Enumerated Constant : simulink/Sources/Enumerated Constant  OutDataTypeStr=Enum: ParameterM_EeepParaIndexType  Value=ParameterM_EeepParaIndexType.PARAMETERM_EEEP_MODEL_TSOC_INDEX  SampleTime=inf
      settings: SourceProductName=Simulink
  S-Function : S-Function  FunctionName=sfn_NVMWrite  SFunctionDeploymentMode=off  EnableBusSupport=off
  Terminator : Terminator
  wires:
  Enumerated Constant/1 -> S-Function/1
  DSOC/1 -> Data Type Conversion/1
  S-Function/1 -> Terminator/1
  Data Type Conversion/1 -> S-Function/2

== system Udan_SOC/SOC_Calculate/UdanSOCCalcn/Subsystem1/Subsystem ==
  HighIndex : Inport
  LowIndex : Inport  Port=2
  Enable : EnablePort
  Add : Sum
  Bit Rotate : hdlsllib/Logic and Bit Operations/Bit Rotate  mode=Rotate Left  N=16
      settings: SourceProductName=HDL Coder  SourceProductBaseCode=HD
  Data Type Conversion : DataTypeConversion  OutDataTypeStr=uint32
  soc : Outport
  wires:
  LowIndex/1 -> Add/2
  Bit Rotate/1 -> Add/1
  Data Type Conversion/1 -> Bit Rotate/1
  HighIndex/1 -> Data Type Conversion/1
  Add/1 -> soc/1  "soc"

== system Udan_SOC/SOC_Calculate/UdanSOCCalcn/WriteOCVTime/Subsystem ==
  data : Inport
  HighIndex : Inport  Port=2
  LowIndex : Inport  Port=3
  Bit Rotate : hdlsllib/Logic and Bit Operations/Bit Rotate  mode=Rotate Right  N=16
      settings: SourceProductName=HDL Coder  SourceProductBaseCode=HD
  Data Type Conversion : DataTypeConversion  OutDataTypeStr=uint16
  Data Type Conversion1 : DataTypeConversion  OutDataTypeStr=uint16
  Logical Operator : Logic  AllPortsSameDT=off  OutDataTypeStr=boolean
  S-Function : S-Function  FunctionName=sfn_NVMWrite  SFunctionDeploymentMode=off  EnableBusSupport=off
  S-Function1 : S-Function  FunctionName=sfn_NVMWrite  SFunctionDeploymentMode=off  EnableBusSupport=off
  WriteResult : Outport
  wires:
  data/1 -> Data Type Conversion1/1, Bit Rotate/1
  Data Type Conversion/1 -> S-Function/2
  Bit Rotate/1 -> Data Type Conversion/1
  Data Type Conversion1/1 -> S-Function1/2
  S-Function/1 -> Logical Operator/1
  HighIndex/1 -> S-Function/1
  LowIndex/1 -> S-Function1/1
  S-Function1/1 -> Logical Operator/2
  Logical Operator/1 -> WriteResult/1

== system Udan_SOC/SOC_Calculate/UdanSOCCalcn/WriteSOH/Enabled Subsystem ==
  index : Inport
  data : Inport  Port=2
  Enable : EnablePort
  S-Function : S-Function  FunctionName=sfn_NVMWrite  SFunctionDeploymentMode=off  EnableBusSupport=off
  EeepWriteFailure : Outport
  wires:
  data/1 -> S-Function/2
  index/1 -> S-Function/1
  S-Function/1 -> EeepWriteFailure/1

== system Udan_SOC/SOC_Calculate/UdanSOCCalcn/WriteSOH/Enabled Subsystem1 ==
  index : Inport
  data : Inport  Port=2
  Enable : EnablePort
  S-Function : S-Function  FunctionName=sfn_NVMWrite  SFunctionDeploymentMode=off  EnableBusSupport=off
  EeepWriteFailure : Outport
  wires:
  data/1 -> S-Function/2
  index/1 -> S-Function/1
  S-Function/1 -> EeepWriteFailure/1

== system Udan_SOC/SOC_Calculate/UdanSOCCalcn/WriteSOH/Enabled Subsystem2 ==
  index : Inport
  data : Inport  Port=2
  Enable : EnablePort
  S-Function : S-Function  FunctionName=sfn_NVMWrite  SFunctionDeploymentMode=off  EnableBusSupport=off
  EeepWriteFailure : Outport
  wires:
  data/1 -> S-Function/2
  index/1 -> S-Function/1
  S-Function/1 -> EeepWriteFailure/1

== system Udan_SOC/SOC_Calculate/UdanSOCCalcn/WriteSOH/Enabled Subsystem3 ==
  index : Inport
  data : Inport  Port=2
  Enable : EnablePort
  S-Function : S-Function  FunctionName=sfn_NVMWrite  SFunctionDeploymentMode=off  EnableBusSupport=off
  EeepWriteFailure : Outport
  wires:
  data/1 -> S-Function/2
  index/1 -> S-Function/1
  S-Function/1 -> EeepWriteFailure/1
